simulink model "ASK"  (R2017a)
settings: Solver=VariableStepAuto  StartTime=0.0  StopTime=10.0  RelTol=1e-3
libraries: commanapbnd3 x2, commchan3 x1, commrandsrc3 x1, simulink x1
settings Model: Creator=81228  LastModifiedBy=81228

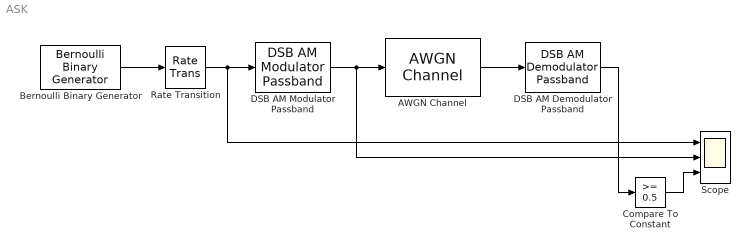
== system ASK ==
  AWGN Channel : commchan3/AWGN Channel  InputProcessing=Columns as channels (frame based)  seed=67  noiseMode="Signal to noise ratio  (Eb/No)"  EbNodB=20  EsNodB=10  SNRdB=10  bitsPerSym=1  Ps=0.001  Tsym=1/500  variance=1
  Bernoulli Binary Generator : commrandsrc3/Bernoulli Binary Generator  ProbabilityOfZero=0.5  SeedSource=Parameter  Seed=12345  SampleTime=1/250  SamplesPerFrame=1  OutputDataType=double  SimulateUsing=Interpreted execution
  Compare To Constant : simulink/Logic and Bit Operations/Compare To Constant  relop=>=  const=0.5  OutDataTypeStr=boolean
  DSB AM Demodulator Passband : commanapbnd3/DSB AM Demodulator Passband  Fc=1000  Ph=0  method=Butterworth  n=4  cf=500  Rp=0.1  Rs=50  Offset=0
      settings: SourceProductName=Communications System Toolbox  SourceProductBaseCode=CM
  DSB AM Modulator Passband : commanapbnd3/DSB AM Modulator Passband  Fc=1000  Ph=0  Offset=0
      settings: SourceProductName=Communications System Toolbox  SourceProductBaseCode=CM
  Rate Transition : RateTransition  OutPortSampleTime=1/10000
  Scope : Scope  NumInputPorts=3
  wires:
  AWGN Channel/1 -> DSB AM Demodulator Passband/1
  DSB AM Modulator Passband/1 -> Scope/2, AWGN Channel/1
  Rate Transition/1 -> Scope/1, DSB AM Modulator Passband/1
  Bernoulli Binary Generator/1 -> Rate Transition/1
  DSB AM Demodulator Passband/1 -> Compare To Constant/1
  Compare To Constant/1 -> Scope/3
